simulink model "scattering_based_bi_teleop_pf_kalman"  (R2020b)
settings: Solver=VariableStepAuto  StartTime=0.0  StopTime=30  RelTol=1e-3
values from neighbouring files (symbols this model uses):
  A = 1    [four_channel_bilateral_teleoperation_kalman_params.m]    (also in four_channel_bilateral_teleoperation_params.m; kalman_test.m = [1 Ts Ts^2/2; 0 1 Ts; 0 0 1]; recursive_estimation.m = [1 Ts Ts^2/2; 0 1 Ts; 0 0 1]; scattering_based_bi_teleop_pf_kalman_params.m)
  b = 1    [scattering_based_bi_teleop_pf_kalman_params.m]    (also in scattering_based_bi_teleop_pf_params.m; scattering_based_bi_teleop_pp_kalman_params.m; scattering_based_bi_teleop_pp_params.m; scattering_based_bilateral_teleoperation_pp_params.m = 0.234)
  Be = 100    [four_channel_bilateral_teleoperation_architecture_params.m]    (also in four_channel_bilateral_teleoperation_kalman_params.m = 0; four_channel_bilateral_teleoperation_params.m = 0; scattering_based_bi_teleop_pf_kalman_params.m = 10; scattering_based_bi_teleop_pf_params.m = 10)
  Bh = 70    [four_channel_bilateral_teleoperation_architecture_params.m]    (also in four_channel_bilateral_teleoperation_kalman_params.m; four_channel_bilateral_teleoperation_params.m; scattering_based_bi_teleop_pf_kalman_params.m = 1.5; scattering_based_bi_teleop_pf_params.m = 1.5)
  Bm = 1    [four_channel_bilateral_teleoperation_architecture_params.m]    (also in four_channel_bilateral_teleoperation_kalman_params.m = 0.8; four_channel_bilateral_teleoperation_params.m = 0.8; scattering_based_bi_teleop_pf_kalman_params.m = 0; scattering_based_bi_teleop_pp_kalman_params.m = 15)
  Bs = 1    [four_channel_bilateral_teleoperation_architecture_params.m]    (also in four_channel_bilateral_teleoperation_kalman_params.m = 3.2; four_channel_bilateral_teleoperation_params.m = 3.2; scattering_based_bi_teleop_pf_kalman_params.m = 40; scattering_based_bi_teleop_pf_params.m = 3)
  delay = 1    [scattering_based_bi_teleop_pf_kalman_params.m]    (also in scattering_based_bi_teleop_pf_params.m; scattering_based_bi_teleop_pp_kalman_params.m; scattering_based_bi_teleop_pp_params.m; tank_based_bi_teleop_pf_kalman.m)
  Dm = 5    [four_channel_bilateral_teleoperation_architecture_params.m]    (also in four_channel_bilateral_teleoperation_kalman_params.m = 0; four_channel_bilateral_teleoperation_params.m = 0; scattering_based_bi_teleop_pf_kalman_params.m = 0; scattering_based_bi_teleop_pf_params.m = 0)
  Ds = 10    [four_channel_bilateral_teleoperation_architecture_params.m]    (also in four_channel_bilateral_teleoperation_kalman_params.m = 0; four_channel_bilateral_teleoperation_params.m = 0; scattering_based_bi_teleop_pf_kalman_params.m = 0; scattering_based_bi_teleop_pf_params.m = 0)
  Fc = 1    [four_channel_bilateral_teleoperation_kalman_params.m]    (also in four_channel_bilateral_teleoperation_params.m; kalman_test.m = 10; scattering_based_bi_teleop_pf_kalman_params.m = 0.1; scattering_based_bi_teleop_pf_params.m)
  Filter = 100    [scattering_based_bi_teleop_pf_kalman_params.m]    (also in scattering_based_bi_teleop_pf_params.m = 5; scattering_based_bi_teleop_pp_kalman_params.m = 10; scattering_based_bi_teleop_pp_params.m = 10; tank_based_bi_teleop_pf_kalman.m)
  Fip = 1    [four_channel_bilateral_teleoperation_kalman_params.m]    (also in four_channel_bilateral_teleoperation_params.m; scattering_based_bi_teleop_pf_kalman_params.m = 5; scattering_based_bi_teleop_pf_params.m; scattering_based_bi_teleop_pp_kalman_params.m = 5)
  Ih = 2    [scattering_based_bi_teleop_pf_kalman_params.m]    (also in scattering_based_bi_teleop_pp_kalman_params.m; scattering_based_bi_teleop_pp_params.m; tank_based_bi_teleop_pf_kalman.m; tank_based_bi_teleop_pf_params.m)
  Je = 0    [four_channel_bilateral_teleoperation_architecture_params.m]    (also in four_channel_bilateral_teleoperation_kalman_params.m; four_channel_bilateral_teleoperation_params.m; scattering_based_bi_teleop_pf_kalman_params.m; scattering_based_bi_teleop_pf_params.m)
  Jh = 0.5    [four_channel_bilateral_teleoperation_architecture_params.m]    (also in four_channel_bilateral_teleoperation_kalman_params.m; four_channel_bilateral_teleoperation_params.m; scattering_based_bi_teleop_pf_kalman_params.m = 0; scattering_based_bi_teleop_pf_params.m = 0.05)
  Ke = 200    [four_channel_bilateral_teleoperation_architecture_params.m]    (also in four_channel_bilateral_teleoperation_kalman_params.m = 50; four_channel_bilateral_teleoperation_params.m = 50; scattering_based_bi_teleop_pf_kalman_params.m; scattering_based_bi_teleop_pf_params.m)
  Kh = 2000    [four_channel_bilateral_teleoperation_architecture_params.m]    (also in four_channel_bilateral_teleoperation_kalman_params.m; four_channel_bilateral_teleoperation_params.m; scattering_based_bi_teleop_pf_kalman_params.m = 1; scattering_based_bi_teleop_pf_params.m = 0)
  Km = 1    [four_channel_bilateral_teleoperation_architecture_params.m]    (also in four_channel_bilateral_teleoperation_kalman_params.m; four_channel_bilateral_teleoperation_params.m; scattering_based_bi_teleop_pf_kalman_params.m = 0; scattering_based_bi_teleop_pp_kalman_params.m = 10)
  Ks = 1    [four_channel_bilateral_teleoperation_architecture_params.m]    (also in four_channel_bilateral_teleoperation_kalman_params.m = 4; four_channel_bilateral_teleoperation_params.m = 4; scattering_based_bi_teleop_pf_kalman_params.m = 50; scattering_based_bi_teleop_pf_params.m = 110)
  Mm = 0.5    [four_channel_bilateral_teleoperation_architecture_params.m]    (also in four_channel_bilateral_teleoperation_kalman_params.m; four_channel_bilateral_teleoperation_params.m; scattering_based_bi_teleop_pf_kalman_params.m; scattering_based_bi_teleop_pf_params.m)
  Ms = 2    [four_channel_bilateral_teleoperation_architecture_params.m]    (also in four_channel_bilateral_teleoperation_kalman_params.m; four_channel_bilateral_teleoperation_params.m; scattering_based_bi_teleop_pf_kalman_params.m; scattering_based_bi_teleop_pf_params.m)
  Ph = 2000    [four_channel_bilateral_teleoperation_kalman_params.m]    (also in four_channel_bilateral_teleoperation_params.m = 50500; scattering_based_bi_teleop_pf_kalman_params.m = 5; scattering_based_bi_teleop_pf_params.m = 23; scattering_based_bi_teleop_pp_kalman_params.m = 6)
  Ts = 0.001    [four_channel_bilateral_teleoperation_kalman_params.m]    (also in four_channel_bilateral_teleoperation_params.m; kalman_test.m; recursive_estimation.m; scattering_based_bi_teleop_pf_kalman_params.m)
  VarianceForces = 0.01    [four_channel_bilateral_teleoperation_kalman_params.m]    (also in four_channel_bilateral_teleoperation_params.m; scattering_based_bi_teleop_pf_kalman_params.m; scattering_based_bi_teleop_pp_kalman_params.m; scattering_based_bi_teleop_pp_params.m)
  VarianceVelocities = 0.001    [four_channel_bilateral_teleoperation_kalman_params.m]    (also in four_channel_bilateral_teleoperation_params.m; scattering_based_bi_teleop_pf_kalman_params.m = 1e-05; scattering_based_bi_teleop_pp_kalman_params.m = 1e-05; scattering_based_bi_teleop_pp_params.m = 1e-05)
undefined symbols (not defined in the file or in its folder): DiscIntNeverNeededParam
settings Model: Creator=anuj  LastModifiedBy=filippo

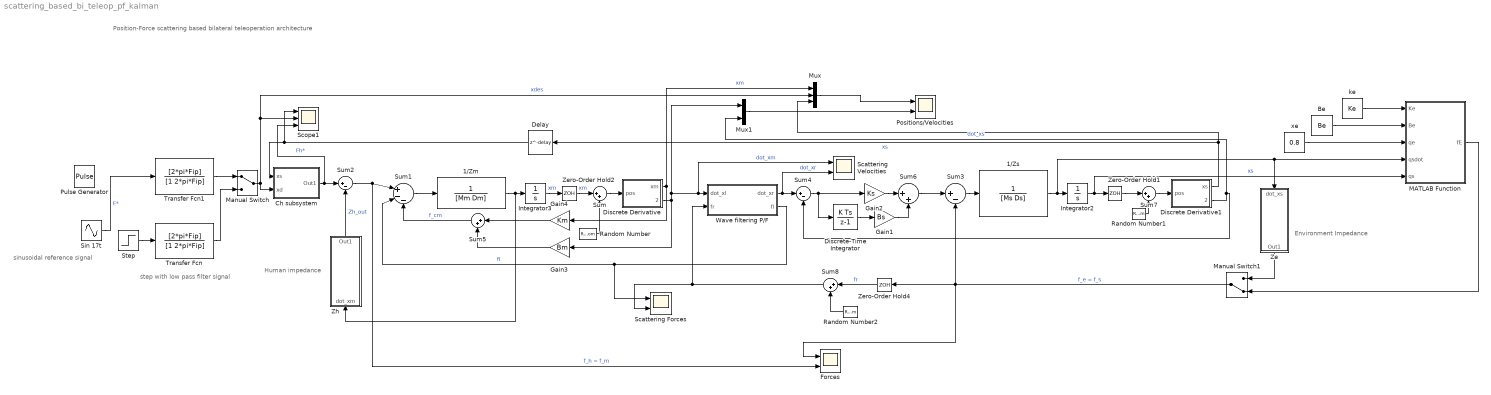
== system scattering_based_bi_teleop_pf_kalman ==
  note: Position-Force scattering based bilateral teleoperation architecture
  note: Environment Impedance
  note: Human impedance
  note: sinusoidal reference signal
  note: step with low pass filter signal
  1/Zm : TransferFcn  Denominator=[Mm Dm]
  1/Zs : TransferFcn  Denominator=[Ms Ds]
  Be : Constant  Value=Be
  Ch subsystem : Subsystem
  Delay : Delay  DelayLength=delay  SampleTime=Ts
  Discrete Derivative : Subsystem
  Discrete Derivative1 : Subsystem
  Discrete-Time Integrator : DiscreteIntegrator  SampleTime=-1  ICPrevOutput=DiscIntNeverNeededParam  ICPrevScaledInput=DiscIntNeverNeededParam
  Forces : Scope  NumInputPorts=2
  Gain1 : Gain  Gain=Bs
  Gain2 : Gain  Gain=Ks
  Gain3 : Gain  Gain=Bm
  Gain4 : Gain  Gain=Km
  Integrator2 : Integrator
  Integrator3 : Integrator
  MATLAB Function : MATLAB Function  TreatAsAtomicUnit=on
  Manual Switch : ManualSwitch
  Manual Switch1 : ManualSwitch  CurrentSetting=0
  Mux : Mux  Inputs=3
  Mux1 : Mux  Inputs=2
  Positions/Velocities : Scope  NumInputPorts=2
  Pulse Generator : DiscretePulseGenerator  PulseType=Time based  Amplitude=A  PulseWidth=50  PhaseDelay=1
  Random Number : RandomNumber  Variance=VarianceVelocities  SampleTime=Ts
  Random Number1 : RandomNumber  Variance=VarianceVelocities  SampleTime=Ts
  Random Number2 : RandomNumber  Variance=VarianceForces  SampleTime=Ts
  Scattering Forces : Scope  NumInputPorts=2
  Scattering Velocities : Scope  NumInputPorts=2
  Scope1 : Scope  NumInputPorts=3
  Sin 17t : Sin  Amplitude=A  Frequency=2*pi*Fc  SampleTime=0
  Step : Step  After=A  SampleTime=0
  Sum{,5..8} (5 alike) : Sum  Inputs=|++
  Sum1 : Sum  Inputs=|+--
  Sum2 : Sum  Inputs=|+-
  Sum3 : Sum  Inputs=|+-
  Sum4 : Sum  Inputs=|+-
  Transfer Fcn : TransferFcn  Numerator=[2*pi*Fip]  Denominator=[1 2*pi*Fip]
  Transfer Fcn1 : TransferFcn  Numerator=[2*pi*Fip]  Denominator=[1 2*pi*Fip]
  Wave filtering P/F : Subsystem
  Ze : Subsystem
  Zero-Order Hold1 : ZeroOrderHold  SampleTime=Ts
  Zero-Order Hold2 : ZeroOrderHold  SampleTime=Ts
  Zero-Order Hold4 : ZeroOrderHold  SampleTime=Ts
  Zh : Subsystem
  ke : Constant  Value=Ke
  xe : Constant  Value=0.8
  wires:
  Sum2/1 -> Forces/2, Sum1/1  "f_h = f_m"
  1/Zm/1 -> Zh/1(dot_xm), Integrator3/1
  Sum1/1 -> 1/Zm/1
  Wave filtering P/F/2(fl) -> Sum1/2, Scattering Forces/1  "fl"
  Sum3/1 -> 1/Zs/1
  Manual Switch1/1 -> Forces/1, Zero-Order Hold4/1, Sum3/2  "f_e = f_s"
  Be/1 -> MATLAB Function/2(Be)
  xe/1 -> MATLAB Function/3(qe)
  ke/1 -> MATLAB Function/1(Ke)
  Transfer Fcn/1 -> Manual Switch/2
  Step/1 -> Transfer Fcn/1
  Zh/1(Out1) -> Sum2/2  "Zh_out"
  Discrete Derivative1/2(dot_xs) -> Sum4/2, Mux1/2  "dot_xs"
  1/Zs/1 -> Integrator2/1, Ze/1(dot_xs), MATLAB Function/4(qsdot)
  Integrator2/1 -> Zero-Order Hold1/1, MATLAB Function/5(qs)  "xs"
  Zero-Order Hold1/1 -> Sum7/1
  Integrator3/1 -> Zero-Order Hold2/1  "xm"
  Discrete Derivative/2(dot_xm) -> Mux1/1, Scattering Velocities/1, Wave filtering P/F/1(dot_xl), Gain3/1  "dot_xm"
  Zero-Order Hold2/1 -> Sum/1  "xm"
  Ze/1(Out1) -> Manual Switch1/1
  MATLAB Function/1(fE) -> Manual Switch1/2
  Mux1/1 -> Positions/Velocities/2
  Mux/1 -> Positions/Velocities/1
  Manual Switch/1 -> Mux/2, Scope1/2, Ch subsystem/2(xd)  "xdes"
  Ch subsystem/1(Out1) -> Scope1/3, Sum2/1  "Fh*"
  Sum6/1 -> Sum3/1
  Gain1/1 -> Sum6/2
  Gain2/1 -> Sum6/1
  Discrete-Time Integrator/1 -> Gain1/1
  Wave filtering P/F/1(dot_xr) -> Sum4/1, Scattering Velocities/2  "dot_xr"
  Sum4/1 -> Discrete-Time Integrator/1, Gain2/1
  Gain4/1 -> Sum5/1
  Sum5/1 -> Sum1/3  "f_cm"
  Gain3/1 -> Sum5/2
  Transfer Fcn1/1 -> Manual Switch/1
  Delay/1 -> Scope1/1, Ch subsystem/1(xs)
  Sum8/1 -> Scattering Forces/2, Wave filtering P/F/2(fr)
  Zero-Order Hold4/1 -> Sum8/1  "fr"
  Sum7/1 -> Discrete Derivative1/1(pos)
  Sum/1 -> Discrete Derivative/1(pos)
  Discrete Derivative/1(xm) -> Gain4/1, Mux/1  "xm"
  Discrete Derivative1/1(xs) -> Delay/1, Mux/3  "xs"
  Random Number2/1 -> Sum8/2
  Random Number/1 -> Sum/2
  Random Number1/1 -> Sum7/2
  Sin 17t/1 -> Transfer Fcn1/1  "F*"

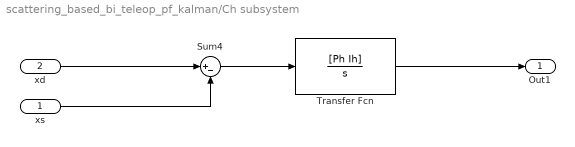
== system scattering_based_bi_teleop_pf_kalman/Ch subsystem ==
  xs : Inport
  xd : Inport  Port=2
  Sum4 : Sum  Inputs=|+-
  Transfer Fcn : TransferFcn  Numerator=[Ph Ih]  Denominator=[1 0]
  Out1 : Outport
  wires:
  xs/1 -> Sum4/2
  Sum4/1 -> Transfer Fcn/1
  Transfer Fcn/1 -> Out1/1
  xd/1 -> Sum4/1

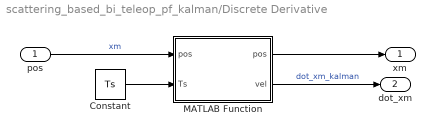
== system scattering_based_bi_teleop_pf_kalman/Discrete Derivative ==
  pos : Inport
  Constant : Constant  Value=Ts
  MATLAB Function : MATLAB Function  TreatAsAtomicUnit=on
  xm : Outport
  dot_xm : Outport  Port=2
  wires:
  pos/1 -> MATLAB Function/1("pos ")  "xm"
  Constant/1 -> MATLAB Function/2(Ts)
  MATLAB Function/1(pos) -> xm/1
  MATLAB Function/2(vel) -> dot_xm/1  "dot_xm_kalman"

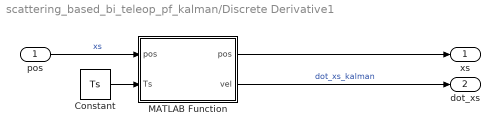
== system scattering_based_bi_teleop_pf_kalman/Discrete Derivative1 ==
  pos : Inport
  Constant : Constant  Value=Ts
  MATLAB Function : MATLAB Function  TreatAsAtomicUnit=on
  xs : Outport
  dot_xs : Outport  Port=2
  wires:
  pos/1 -> MATLAB Function/1("pos ")  "xs"
  Constant/1 -> MATLAB Function/2(Ts)
  MATLAB Function/1(pos) -> xs/1
  MATLAB Function/2(vel) -> dot_xs/1  "dot_xs_kalman"

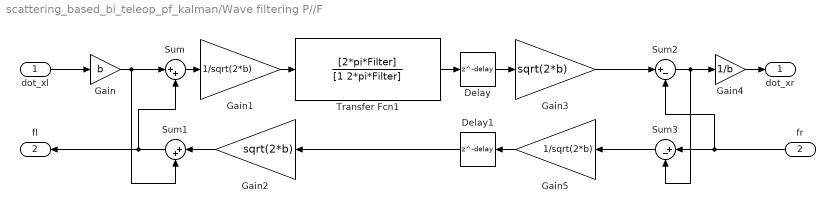
== system scattering_based_bi_teleop_pf_kalman/Wave filtering P//F ==
  dot_xl : Inport
  fr : Inport  Port=2
  Delay : Delay  DelayLength=delay  SampleTime=Ts
  Delay1 : Delay  DelayLength=delay  SampleTime=Ts
  Gain : Gain  Gain=b
  Gain1 : Gain  Gain=1/sqrt(2*b)
  Gain2 : Gain  Gain=sqrt(2*b)
  Gain3 : Gain  Gain=sqrt(2*b)
  Gain4 : Gain  Gain=1/b
  Gain5 : Gain  Gain=1/sqrt(2*b)
  Sum : Sum  Inputs=|++
  Sum1 : Sum  Inputs=|++
  Sum2 : Sum  Inputs=|+-
  Sum3 : Sum  Inputs=|+-
  Transfer Fcn1 : TransferFcn  Numerator=[2*pi*Filter]  Denominator=[1 2*pi*Filter]
  dot_xr : Outport
  fl : Outport  Port=2
  wires:
  Sum2/1 -> Sum3/2, Gain4/1
  Gain/1 -> Sum1/2, Sum/1
  Sum/1 -> Gain1/1
  Gain2/1 -> Sum1/1
  fr/1 -> Sum2/2, Sum3/1
  Sum3/1 -> Gain5/1
  Gain3/1 -> Sum2/1
  Delay/1 -> Gain3/1
  dot_xl/1 -> Gain/1
  Gain4/1 -> dot_xr/1
  Sum1/1 -> fl/1, Sum/2
  Delay1/1 -> Gain2/1
  Gain5/1 -> Delay1/1
  Gain1/1 -> Transfer Fcn1/1
  Transfer Fcn1/1 -> Delay/1

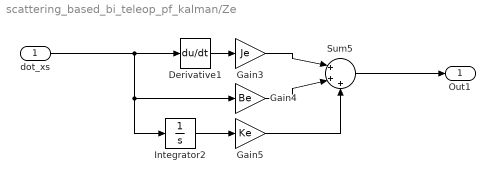
== system scattering_based_bi_teleop_pf_kalman/Ze ==
  dot_xs : Inport
  Derivative1 : Derivative
  Gain3 : Gain  Gain=Je
  Gain4 : Gain  Gain=Be
  Gain5 : Gain  Gain=Ke
  Integrator2 : Integrator
  Sum5 : Sum  Inputs=|+++
  Out1 : Outport
  wires:
  Gain4/1 -> Sum5/2
  Gain3/1 -> Sum5/1
  Gain5/1 -> Sum5/3
  Sum5/1 -> Out1/1
  Integrator2/1 -> Gain5/1
  dot_xs/1 -> Integrator2/1, Gain4/1, Derivative1/1
  Derivative1/1 -> Gain3/1

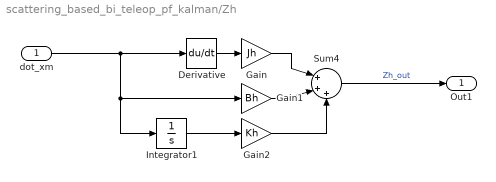
== system scattering_based_bi_teleop_pf_kalman/Zh ==
  dot_xm : Inport
  Derivative : Derivative
  Gain : Gain  Gain=Jh
  Gain1 : Gain  Gain=Bh
  Gain2 : Gain  Gain=Kh
  Integrator1 : Integrator
  Sum4 : Sum  Inputs=|+++
  Out1 : Outport
  wires:
  Derivative/1 -> Gain/1
  Integrator1/1 -> Gain2/1
  Gain2/1 -> Sum4/3
  Gain1/1 -> Sum4/2
  Gain/1 -> Sum4/1
  Sum4/1 -> Out1/1  "Zh_out"
  dot_xm/1 -> Gain1/1, Integrator1/1, Derivative/1

== matlab function scattering_based_bi_teleop_pf_kalman/Discrete Derivative/MATLAB Function ==
  data: pos output; pos input; vel output; Ts input
function [pos, vel] = kalman(pos, Ts)
    persistent P A C Q R x_filter_old P_filter_old
    if isempty(P)
        P = 0;
        x_filter_old=[pos; 0];
        P_filter_old=0.1*eye(2);
        A=[1 Ts; 0 1];
        C=[1 0];
        q=1000000;
        Q=q*[Ts^2/2;Ts]*[Ts^2/2;Ts]';
        R=1;
    end

    % Prediction step (A priori estimation)
    x_kplus1_k = A*x_filter_old;
    P_kplus1_k = A*P_filter_old*A'+Q;

    % Compute the kalman gain
    K = P_kplus1_k * C' * inv(C * P_kplus1_k * C' + R);

    % Calculate the estimation step
    x_kplus1_kplus1 = x_kplus1_k + K *(pos - C * x_kplus1_k);
    P_kplus1_kplus1 = P_kplus1_k - P_kplus1_k * C' * inv(C * P_kplus1_k * C' + R) * C * P_kplus1_k;
    
    % Next step iteration
    x_filter_old = x_kplus1_kplus1;
    P_filter_old = P_kplus1_kplus1;
    
    pos = x_kplus1_kplus1(1,:);
    vel = x_kplus1_kplus1(2,:);
end

== matlab function scattering_based_bi_teleop_pf_kalman/MATLAB Function ==
  data: Ke input; fE output; Be input; qe input; qsdot input; qs input
function fE = environment(Ke, Be, qe, qsdot, qs)
    if qs > qe
        fE = Ke * (qs - qe) + Be * qsdot; % Plot both contributions Ke and Be
    else
        fE = 0;
    end
end

== matlab function scattering_based_bi_teleop_pf_kalman/Discrete Derivative1/MATLAB Function ==
  data: pos output; pos input; vel output; Ts input
function [pos, vel] = kalman(pos, Ts)
    persistent P A C Q R x_filter_old P_filter_old
    if isempty(P)
        P = 0;
        x_filter_old=[pos; 0];
        P_filter_old=0.1*eye(2);
        A=[1 Ts; 0 1];
        C=[1 0];
        q=1000000;
        Q=q*[Ts^2/2;Ts]*[Ts^2/2;Ts]';
        R=1;
    end

    % Prediction step (A priori estimation)
    x_kplus1_k = A*x_filter_old;
    P_kplus1_k = A*P_filter_old*A'+Q;

    % Compute the kalman gain
    K = P_kplus1_k * C' * inv(C * P_kplus1_k * C' + R);

    % Calculate the estimation step
    x_kplus1_kplus1 = x_kplus1_k + K *(pos - C * x_kplus1_k);
    P_kplus1_kplus1 = P_kplus1_k - P_kplus1_k * C' * inv(C * P_kplus1_k * C' + R) * C * P_kplus1_k;
    
    % Next step iteration
    x_filter_old = x_kplus1_kplus1;
    P_filter_old = P_kplus1_kplus1;
    
    pos = x_kplus1_kplus1(1,:);
    vel = x_kplus1_kplus1(2,:);
end
